simulink model "model"  (R2012b)
settings: Solver=ode45  StartTime=0.0  StopTime=.5  RelTol=1e-3
undefined symbols (not defined in the file): A, j
libraries: simulink x1
settings Model: Creator=hamid  LastModifiedBy=hamid

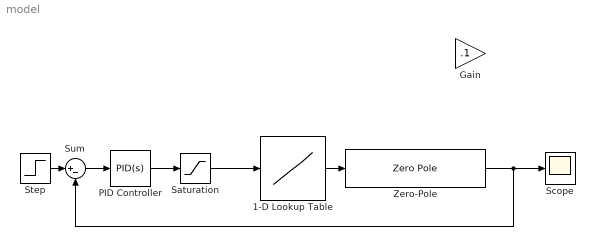
== system model ==
  1-D Lookup Table : Lookup_n-D  NumberOfTableDimensions=1  BreakpointsForDimension1=A(:,1)  Table=A(:,3)  InterpMethod=Cubic spline  ExtrapMethod=Clip  RndMeth=Simplest  InputSameDT=on
  Gain : Gain  Gain=.1  SampleTime=1e-5
  PID Controller : simulink/Continuous/PID Controller  Controller=PID  TimeDomain=Continuous-time  SampleTime=1  IntegratorMethod=Forward Euler  FilterMethod=Forward Euler  Form=Parallel  P=4  I=0  D=0  N=100  InitialConditionSource=internal  InitialConditionForIntegrator=0  InitialConditionForFilter=0  ExternalReset=none  LimitOutput=off  UpperSaturationLimit=inf  LowerSaturationLimit=-inf  LinearizeAsGain=on  AntiWindupMode=none  Kb=1  TrackingMode=off  Kt=1  PParamMin=[]  PParamMax=[]  IParamMin=[]  IParamMax=[]  DParamMin=[]  DParamMax=[]  NParamMin=[]  NParamMax=[]  KbParamMin=[]  KbParamMax=[]  KtParamMin=[]  KtParamMax=[]  POutMin=[]  POutMax=[]  IOutMin=[]  IOutMax=[]  DOutMin=[]  DOutMax=[]  NOutMin=[]  NOutMax=[]  KbOutMin=[]  KbOutMax=[]  KtOutMin=[]  KtOutMax=[]  IntegratorOutMin=[]  IntegratorOutMax=[]  FilterOutMin=[]  FilterOutMax=[]  SumOutMin=[]  SumOutMax=[]  SumI1OutMin=[]  SumI1OutMax=[]  SumI2OutMin=[]  SumI2OutMax=[]  SumI3OutMin=[]  SumI3OutMax=[]  SumDOutMin=[]  SumDOutMax=[]  SaturationOutMin=[]  SaturationOutMax=[]  IntegratorContinuousStateAttributes=''  IntegratorStateMustResolveToSignalObject=off  IntegratorRTWStateStorageClass=Auto  FilterContinuousStateAttributes=''  FilterStateMustResolveToSignalObject=off  FilterRTWStateStorageClass=Auto
  Saturation : Saturate  UpperLimit=.4  LowerLimit=-0.4
  Scope : Scope
      settings: TimeRange=0.5  YMin=0  YMax=0.12
  Step : Step  Time=.1  After=.1  SampleTime=0
  Sum : Sum  Inputs=|+-
  Zero-Pole : ZeroPole  Zeros=[]  Poles=[-1e3+j*1e2 -1e3-j*1e2]  Gain=(-1e3+j*1e2)*(-1e3-j*1e2)
  wires:
  1-D Lookup Table/1 -> Zero-Pole/1
  Sum/1 -> PID Controller/1
  Step/1 -> Sum/1
  PID Controller/1 -> Saturation/1
  Zero-Pole/1 -> Sum/2, Scope/1
  Saturation/1 -> 1-D Lookup Table/1
